simulink model "MotorController_Motor"  (R2020a)
settings: Solver=VariableStepAuto  StartTime=0.0  StopTime=10.0  RelTol=1e-3
libraries: autolibmotorctrlr x1, autolibpmsminterior x1
settings Model: Creator=Administrator  LastModifiedBy=Administrator

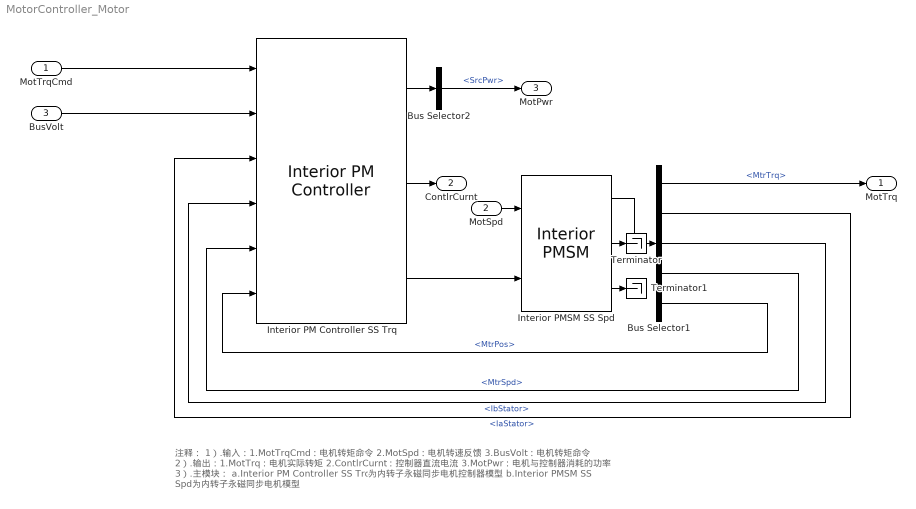
== system MotorController_Motor ==
  note: 注释：
      | 1）.输入：1.MotTrqCmd：电机转矩命令
      | 2.MotSpd：电机转速反馈
      | 3.BusVolt：电机转矩命令
      | 2）.输出：1.MotTrq：电机实际转矩
      | 2.ContlrCurnt：控制器直流电流
      | 3.MotPwr：电机与控制器消耗的功率
      | 3）.主模块：
      | a.Interior PM Controller SS Trq为内转子永磁同步电机控制器模型
      | b.Interior PMSM SS Spd为内转子永磁同步电机模型
  MotTrqCmd : Inport
  MotSpd : Inport  Port=2
  BusVolt : Inport  Port=3
  Bus Selector1 : BusSelector  OutputSignals=MtrTrq,IaStator,IbStator,MtrSpd,MtrPos
  Bus Selector2 : BusSelector  OutputSignals=SrcPwr
  Interior PM Controller SS Trq : autolibmotorctrlr/Interior PM Controller  control_type=Torque Control  Rs=6e-3  Ld=52e-6  Lq=56e-6  lambda_pm=0.0257  PolePairs=10  Mechanical=Mechanical  T_max=140  bp=10  T_mtpa=[0 15.531226878328 31.0642852747721 46.6010049095523 62.1432119156802 77.6927270667208 93.2513640299298 108.820927652792 124.403212290623 140.000000182471]  id_mtpa=[0 -0.252602944280072 -1.01017357706881 -2.27199841989307 -4.03689206860216 -6.30320274051235 -9.06881995564731 -12.3311842693036 -16.0872989522962 -20.3337434963309]  iq_mtpa=[0 40.2869423665694 80.5691360467715 120.841846330784 161.100366350739 201.340030725588 241.556228879371 281.744417931854 321.900135066892 362.019009291639]  idq_limits=[-20.333741947309 362.019009378644 362.589608528808]  EV_current=400  Tst=5e-5  Kp_d=0.13069  Kp_q=0.14074  Ki=15.0796  EV_motion=EV_motion  EV_sf=EV_sf  ba=ba  Ksa=Ksa  Kisa=Kisa  Ksf=Ksf  Jcomp=Jcomp  Fv=Fv  Fs=Fs  param_loss=Single efficiency measurement  eff=98  w_loss_bp=[0 200 400 600 800 1000]  T_loss_bp=[0 25 50 75 100]  losses_table=[100 100 100 100 100;100 150 200 250 300;100 200 300 400 500;100 250 400 550 700;100 300 500 700 900;100 350 600 850 1100]  w_eff_bp=[200 400 600 800 1000]  T_eff_bp=[25 50 75 100]  efficiency_table=[96.2 98.1 98.7 99;98.1 99 99.4 99.5;98.7 99.4 99.6 99.7;99 99.5 99.7 99.8;99.2 99.6 99.7 99.8]  x_w_bp=[-1000 -800 -600 -400 -200 200 400 600 800 1000]  x_T_bp=[-100 -75 -50 -25 25 50 75 100]  x_losses_mat=[200.400801603196 225.67703109328 200.803212851408 201.612903225806 199.999999999997 200 225 200;160.320641282556 180.541624874624 201.005025125625 202.020202020203 200 200 180 160;180.541624874624 180.722891566267 181.086519114686 197.568389057748 194.999999999999 179.999999999997 180 180;201.005025125625 181.086519114686 202.020202020203 193.67991845056 190 200 179.999999999997 200;202.020202020203 197.568389057748 193.67991845056 197.505197505197 190 190 194.999999999999 200;200 194.999999999999 190 190 197.505197505197 193.67991845056 197.568389057748 202.020202020203;200 179.999999999997 200 190 193.67991845056 202.020202020203 181.086519114686 201.005025125625;180 180 179.999999999997 194.999999999999 197.568389057748 181.086519114686 180.722891566267 180.541624874624;160 180 200 200 202.020202020203 201.005025125625 180.541624874624 160.320641282556;200 225 200 199.999999999997 201.612903225806 200.803212851408 225.67703109328 200.400801603196]  Tsm=5e-4
      settings: SourceProductBaseCode=PW
  Interior PMSM SS Spd : autolibpmsminterior/Interior PMSM  port_config=Speed  sim_type=Continuous  Ts=0  P=10  Rs=6e-3  Ldq=[52e-6, 56e-6]  KConstText=Permanent flux linkage constant (lambda_pm):  lambda_pm=0.0257  Ke=159.9771  mechanical=[0.023,0,0.5]  idq0=[0,0]  theta_init=0  omega_init=0  KConst=0.0257  lambda_pm_calc=0.0257  Kt=1.323  RefBlkName=autolibpmsmexterior/Surface Mount PMSM  aMode=1
      settings: SourceProductBaseCode=PW
  Terminator : Terminator
  Terminator1 : Terminator
  MotTrq : Outport  VectorParamsAs1DForOutWhenUnconnected=off
  ContlrCurnt : Outport  Port=2  VectorParamsAs1DForOutWhenUnconnected=off
  MotPwr : Outport  Port=3  VectorParamsAs1DForOutWhenUnconnected=off
  wires:
  Interior PM Controller SS Trq/2 -> ContlrCurnt/1
  Bus Selector2/1 -> MotPwr/1  "<SrcPwr>"
  Interior PM Controller SS Trq/1 -> Bus Selector2/1
  BusVolt/1 -> Interior PM Controller SS Trq/2
  Bus Selector1/4 -> Interior PM Controller SS Trq/5  "<MtrSpd>"
  Interior PMSM SS Spd/1 -> Bus Selector1/1
  MotSpd/1 -> Interior PMSM SS Spd/1
  Bus Selector1/3 -> Interior PM Controller SS Trq/4  "<IbStator>"
  MotTrqCmd/1 -> Interior PM Controller SS Trq/1
  Bus Selector1/1 -> MotTrq/1  "<MtrTrq>"
  Interior PM Controller SS Trq/3 -> Interior PMSM SS Spd/2
  Bus Selector1/5 -> Interior PM Controller SS Trq/6  "<MtrPos>"
  Bus Selector1/2 -> Interior PM Controller SS Trq/3  "<IaStator>"
  Interior PMSM SS Spd/2 -> Terminator/1
  Interior PMSM SS Spd/3 -> Terminator1/1
